simulink model "quartercar_freq"  (R2022a)
settings: Solver=VariableStepAuto  StartTime=0.0  StopTime=10  RelTol=1e-3
undefined symbols (not defined in the file): c1, k1, k2, mc, ms
libraries: simulink x1
settings Model: Creator=bjmyn  LastModifiedBy=bjmyn

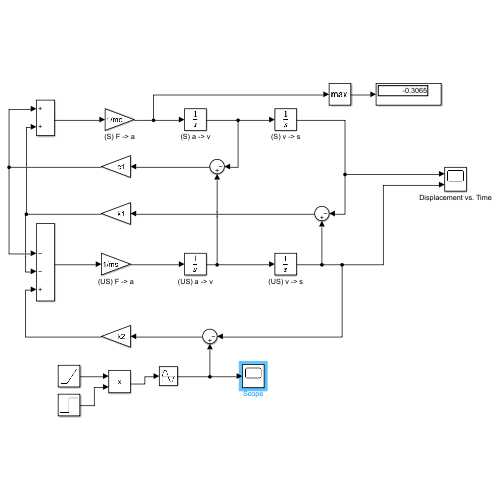
[thumbnail: Simulink's stored preview of the top-level diagram]
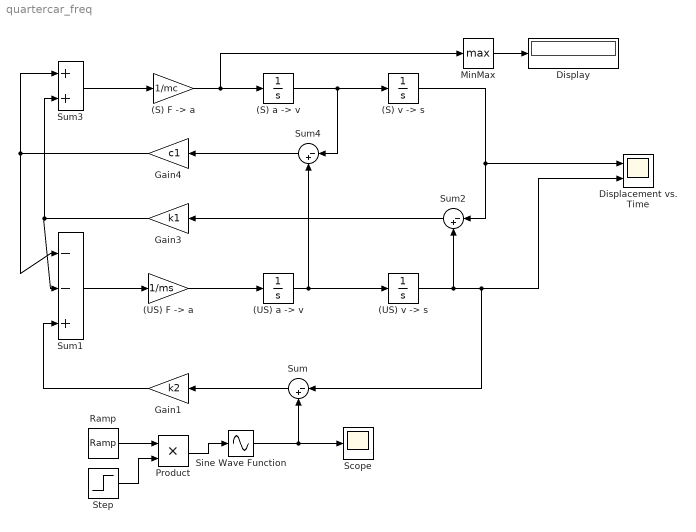
== system quartercar_freq ==
  "(S) F -> a" : Gain  Gain=1/mc
  "(S) a -> v" : Integrator
  "(S) v -> s" : Integrator
  "(US) F -> a" : Gain  Gain=1/ms
  "(US) a -> v" : Integrator
  "(US) v -> s" : Integrator
  Displacement vs. Time : Scope  NumInputPorts=2
  Display : Display
  Gain1 : Gain  Gain=k2
  Gain3 : Gain  Gain=k1
  Gain4 : Gain  Gain=c1
  MinMax : MinMax  Function=max
  Product : Product
  Ramp : simulink/Sources/Ramp  slope=1  start=0  InitialOutput=0
  Scope : Scope
  Sine Wave Function : Sin  TimeSource=Use external signal  Frequency=2*pi  SampleTime=0
  Step : Step  Time=5  Before=5  After=15  SampleTime=0
  Sum : Sum  Inputs=|-+
  Sum1 : Sum  Inputs=|--+
  Sum2 : Sum  Inputs=|-+
  Sum3 : Sum
  Sum4 : Sum  Inputs=|-+
  wires:
  Sine Wave Function/1 -> Scope/1, Sum/2
  Sum/1 -> Gain1/1
  Gain1/1 -> Sum1/3
  Sum1/1 -> "(US) F -> a"/1
  "(US) F -> a"/1 -> "(US) a -> v"/1
  "(US) a -> v"/1 -> Sum4/2, "(US) v -> s"/1
  "(US) v -> s"/1 -> Sum2/2, Displacement vs. Time/2, Sum/1
  "(S) a -> v"/1 -> Sum4/1, "(S) v -> s"/1
  "(S) v -> s"/1 -> Sum2/1, Displacement vs. Time/1
  Sum2/1 -> Gain3/1
  Gain3/1 -> Sum3/2, Sum1/2
  Sum4/1 -> Gain4/1
  Gain4/1 -> Sum1/1, Sum3/1
  Sum3/1 -> "(S) F -> a"/1
  "(S) F -> a"/1 -> MinMax/1, "(S) a -> v"/1
  MinMax/1 -> Display/1
  Ramp/1 -> Product/1
  Product/1 -> Sine Wave Function/1
  Step/1 -> Product/2
